simulink model "ObservadorConIntegrador"  (R2023b)
settings: Solver=VariableStepAuto  StartTime=0.0  StopTime=10.0  RelTol=1e-3
values from neighbouring files (symbols this model uses):
  J_eq = J_m + J_l/(r^2)    (= 4.58263888889e-05)    [varLC.m]
undefined symbols (not defined in the file or in its folder): K_obs_i, K_obs_theta2, K_obs_w2
settings Model: Creator=gonza  LastModifiedBy=tomas

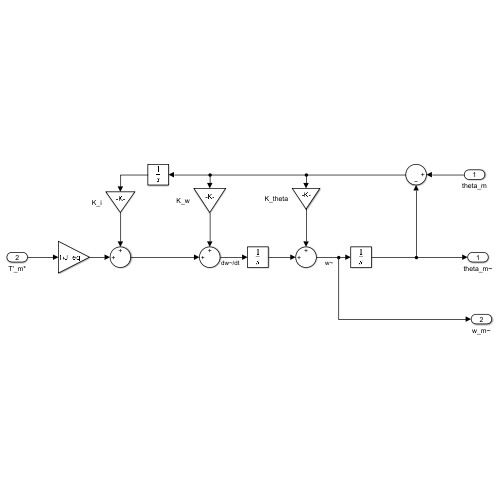
[thumbnail: Simulink's stored preview of the top-level diagram]
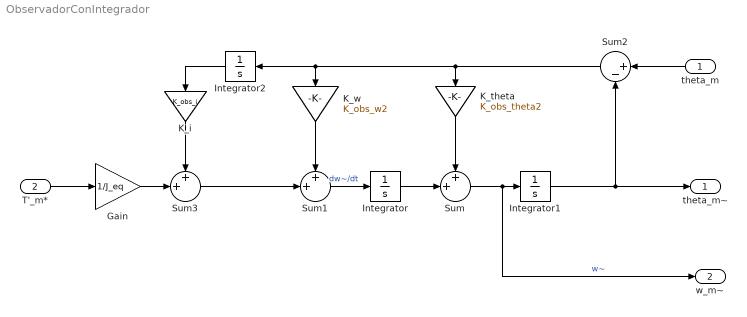
== system ObservadorConIntegrador ==
  theta_m : Inport
  T'_m* : Inport  Port=2
  Gain : Gain  Gain=1/J_eq
  Integrator : Integrator
  Integrator1 : Integrator
  Integrator2 : Integrator
  K_i : Gain  Gain=K_obs_i
  K_theta : Gain  Gain=K_obs_theta2
  K_w : Gain  Gain=K_obs_w2
  Sum : Sum  Inputs=++|
  Sum1 : Sum  Inputs=++|
  Sum2 : Sum  Inputs=|+-
  Sum3 : Sum  Inputs=++|
  theta_m~ : Outport
  w_m~ : Outport  Port=2
  wires:
  T'_m*/1 -> Gain/1
  Integrator1/1 -> theta_m~/1, Sum2/2
  theta_m/1 -> Sum2/1
  K_theta/1 -> Sum/1
  K_w/1 -> Sum1/1
  Sum2/1 -> Integrator2/1, K_w/1, K_theta/1
  Sum1/1 -> Integrator/1  "dw~/dt"
  Integrator/1 -> Sum/2
  Sum/1 -> w_m~/1, Integrator1/1  "w~"
  Gain/1 -> Sum3/2
  Sum3/1 -> Sum1/2
  K_i/1 -> Sum3/1
  Integrator2/1 -> K_i/1
